simulink model "parachute_dynamics_simulink"  (R2024b)
settings: Solver=VariableStepAuto  StartTime=0.0  StopTime=100  RelTol=1e-3
undefined symbols (not defined in the file or in its folder): M_para, parachute_Ixx, parachute_Iyy, parachute_Izz, payload_mass
libraries: shared6dof x1
settings Model: Creator=Venkat Jayadevan  LastModifiedBy=Venkat Jayadevan

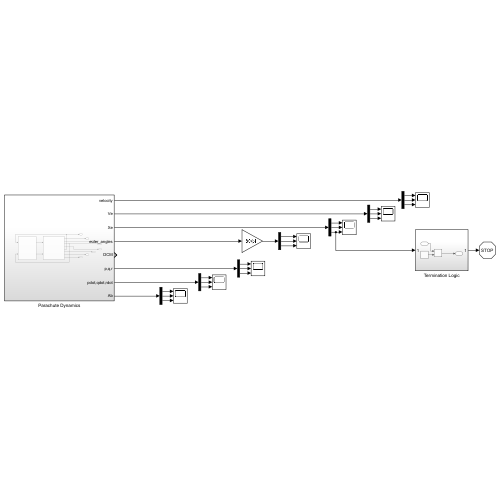
[thumbnail: Simulink's stored preview of the top-level diagram]
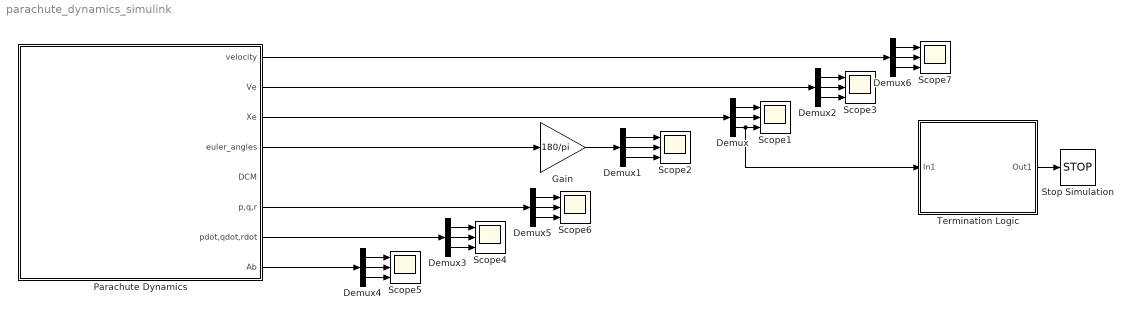
== system parachute_dynamics_simulink ==
  Demux{,1..6} (7 alike) : Demux  Outputs=3
  Gain : Gain  Gain=180/pi
  Parachute Dynamics : Subsystem
  Scope{1..7} (7 alike) : Scope  NumInputPorts=3
  Stop Simulation : Stop
  Termination Logic : Subsystem
  wires:
  Demux/1 -> Scope1/1
  Demux/2 -> Scope1/2
  Demux/3 -> Termination Logic/1(In1), Scope1/3
  Demux1/2 -> Scope2/2
  Demux1/1 -> Scope2/1
  Demux1/3 -> Scope2/3
  Demux2/2 -> Scope3/2
  Demux2/1 -> Scope3/1
  Demux2/3 -> Scope3/3
  Demux3/2 -> Scope4/2
  Demux3/3 -> Scope4/3
  Demux3/1 -> Scope4/1
  Demux5/2 -> Scope6/2
  Demux5/3 -> Scope6/3
  Demux4/1 -> Scope5/1
  Demux4/2 -> Scope5/2
  Demux5/1 -> Scope6/1
  Demux4/3 -> Scope5/3
  Gain/1 -> Demux1/1
  Demux6/1 -> Scope7/1
  Demux6/2 -> Scope7/2
  Demux6/3 -> Scope7/3
  Parachute Dynamics/1(velocity) -> Demux6/1
  Parachute Dynamics/2(Ve) -> Demux2/1
  Parachute Dynamics/3(Xe) -> Demux/1
  Parachute Dynamics/4(euler_angles) -> Gain/1
  Parachute Dynamics/6(p,q,r) -> Demux5/1
  Parachute Dynamics/7(pdot,qdot,rdot) -> Demux3/1
  Parachute Dynamics/8(Ab) -> Demux4/1
  Termination Logic/1(Out1) -> Stop Simulation/1

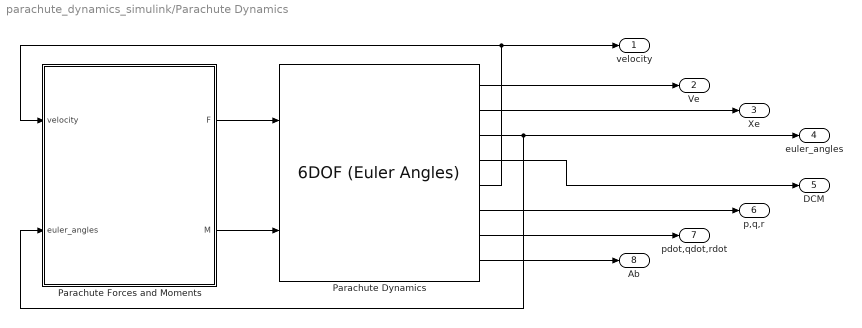
== system parachute_dynamics_simulink/Parachute Dynamics ==
  Parachute Dynamics : shared6dof/6DOF (Euler Angles)  units=Metric (MKS)  mtype=Fixed  rep=Euler Angles  xme_0=[0 0 -5000]  Vm_0=[0 0 30]  eul_0=deg2rad([0 0 0])  pm_0=[0 0 0]  mass_0=M_para+payload_mass  mass_e=0.5  mass_f=2.0  inertia=[parachute_Ixx, 0, 0; 0, parachute_Iyy, 0; 0, 0, parachute_Izz]  inertia_e=eye(3)  inertia_f=2*eye(3)  k_quat=1.0  vre_flag=on  abi_flag=off  aMode=0  xme_statename=''  Vm_statename=''  eul_statename=''  quat_statename=''  pm_statename=''  mass_statename=''
  Parachute Forces and Moments : MATLAB Function  TreatAsAtomicUnit=on
  velocity : Outport
  Ve : Outport  Port=2
  Xe : Outport  Port=3
  euler_angles : Outport  Port=4
  DCM : Outport  Port=5
  p,q,r : Outport  Port=6
  pdot,qdot,rdot : Outport  Port=7
  Ab : Outport  Port=8
  wires:
  Parachute Dynamics/5 -> velocity/1, Parachute Forces and Moments/1(velocity)
  Parachute Dynamics/7 -> pdot,qdot,rdot/1
  Parachute Forces and Moments/2(M) -> Parachute Dynamics/2
  Parachute Dynamics/3 -> euler_angles/1, Parachute Forces and Moments/2(euler_angles)
  Parachute Forces and Moments/1(F) -> Parachute Dynamics/1
  Parachute Dynamics/6 -> p,q,r/1
  Parachute Dynamics/8 -> Ab/1
  Parachute Dynamics/1 -> Ve/1
  Parachute Dynamics/2 -> Xe/1
  Parachute Dynamics/4 -> DCM/1

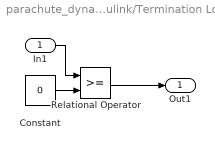
== system parachute_dynamics_simulink/Termination Logic ==
  In1 : Inport
  Constant : Constant  Value=0
  Relational Operator : RelationalOperator  OutDataTypeStr=boolean  RndMeth=Simplest  InputSameDT=off
  Out1 : Outport
  wires:
  Relational Operator/1 -> Out1/1
  Constant/1 -> Relational Operator/2
  In1/1 -> Relational Operator/1

== matlab function parachute_dynamics_simulink/Parachute Dynamics/Parachute Forces and Moments ==
  data: velocity input; euler_angles input; F output; M output
function [F, M] = getForcesAndMoments(velocity, euler_angles)

M_para       =  5832.108;
payload_mass = 69321.000;
density      =     1.225;
g            =     9.806;

z_com_para   =   -81.804;
z_cop_para   =   -89.000;
z_com_payload =   43.280;
z_cop_payload =   43.280;

A_parachute  =   619.276;
A_payload    =    10.000;


phi   = euler_angles(1);
theta = euler_angles(2);
% psi   = euler_angles(3);

u     = velocity(1);
v     = velocity(2);
w     = velocity(3);

    GravityMoment_para_x = M_para*g*cos(theta) * (- z_com_para*sin(phi));
    GravityMoment_para_y = M_para*g*(-z_com_para*sin(theta));
    GravityMoment_para_z = 0 ; % equates to zero because axial symmetry

    % Gravity moment of the payload along x,y and z components
    GravityMoment_payload_x = payload_mass*g*cos(theta)*(- z_com_payload*sin(phi));
    GravityMoment_payload_y = payload_mass*g*(-z_com_payload*sin(theta));
    GravityMoment_payload_z = 0;

    V_total = sqrt(u^2 + v^2 + w^2);

    alpha = acos(w/V_total);

    % Componetize CD and CL into tangential and normal force coefficients
    CT_para = 0.5755 - 0.8091*alpha^2 + 0.4228*alpha^4;
    CN_para = 0.3795*alpha + 0.3631*alpha^3;

    CT_payload = 0.6989 + 12.56*alpha^2 - 35.59*alpha^4;
    CN_payload = 3.645*alpha + 15.20*alpha^3;

    if (u == 0 && v == 0)
        Aerodynamic_force_para_x = 0; Aerodynamic_force_payload_x = 0;
        Aerodynamic_force_para_y = 0; Aerodynamic_force_payload_y = 0;
        Aerodynamic_force_para_z = -0.5*density*CT_para*V_total*V_total*A_parachute; Aerodynamic_force_payload_z = -0.5*density*CT_payload*V_total*V_total*A_payload;
    else
    % Aerodynamic force along x,y,z axes F = 0.5*rho*v^2*A
        Aerodynamic_force_para_x = -0.5*density*CN_para*V_total*V_total*A_parachute*(u/sqrt(u^2 + v^2)); Aerodynamic_force_payload_x = -0.5*density*CN_payload*V_total*V_total*A_payload*(u/sqrt(u^2 + v^2));
        Aerodynamic_force_para_y = -0.5*density*CN_para*V_total*V_total*A_parachute*(v/sqrt(u^2 + v^2)); Aerodynamic_force_payload_y = -0.5*density*CN_payload*V_total*V_total*A_payload*(v/sqrt(u^2 + v^2));
        Aerodynamic_force_para_z = -0.5*density*CT_para*V_total*V_total*A_parachute; Aerodynamic_force_payload_z = -0.5*density*CT_payload*V_total*V_total*A_payload;
    end

    Aerodynamic_moment_x = - z_cop_para*Aerodynamic_force_para_y - z_cop_payload*Aerodynamic_force_payload_y;
    Aerodynamic_moment_y =   z_cop_para*Aerodynamic_force_para_x + z_cop_payload*Aerodynamic_force_payload_x;
    Aerodynamic_moment_z = 0;

    Force_x  = Aerodynamic_force_para_x + Aerodynamic_force_payload_x + (M_para + payload_mass) * g *(-sin(theta));
    Force_y  = Aerodynamic_force_para_y + Aerodynamic_force_payload_y + (M_para + payload_mass) * g * (sin(phi) * cos(theta));
    Force_z  = Aerodynamic_force_para_z + Aerodynamic_force_payload_z + (M_para + payload_mass) * g * (cos(phi) * cos(theta));

    Moment_x = GravityMoment_para_x + GravityMoment_payload_x + Aerodynamic_moment_x;
    Moment_y = GravityMoment_para_y + GravityMoment_payload_y + Aerodynamic_moment_y;
    Moment_z = GravityMoment_para_z + GravityMoment_payload_z + Aerodynamic_moment_z;

    F = [ Force_x;  Force_y;  Force_z];
    M = [Moment_x; Moment_y; Moment_z];
end
